simulink model "inverted_pendulum_2dof"  (R2021b)
settings: Solver=ode45  StartTime=0.0  StopTime=10.0  RelTol=1e-3
undefined symbols (not defined in the file): d, F, g, L, M, m, o_0, t_0, v_0, x_0
settings Model: Creator=lenna  LastModifiedBy=lenna

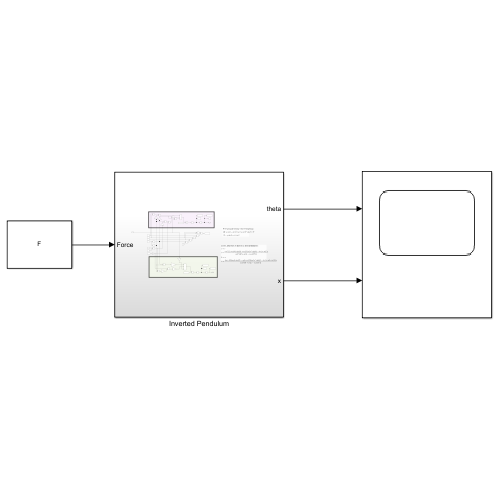
[thumbnail: Simulink's stored preview of the top-level diagram]
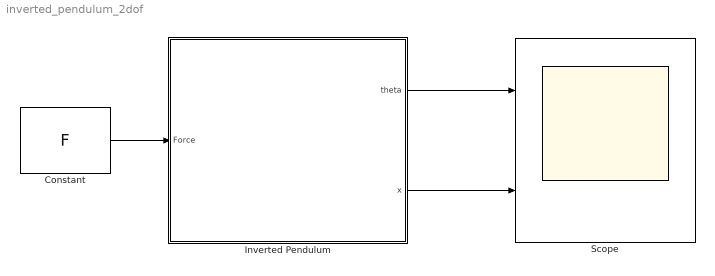
== system inverted_pendulum_2dof ==
  Constant : Constant  Value=F
  Inverted Pendulum : Subsystem
  Scope : Scope  NumInputPorts=2
  wires:
  Constant/1 -> Inverted Pendulum/1(Force)
  Inverted Pendulum/1(theta) -> Scope/1
  Inverted Pendulum/2(x) -> Scope/2

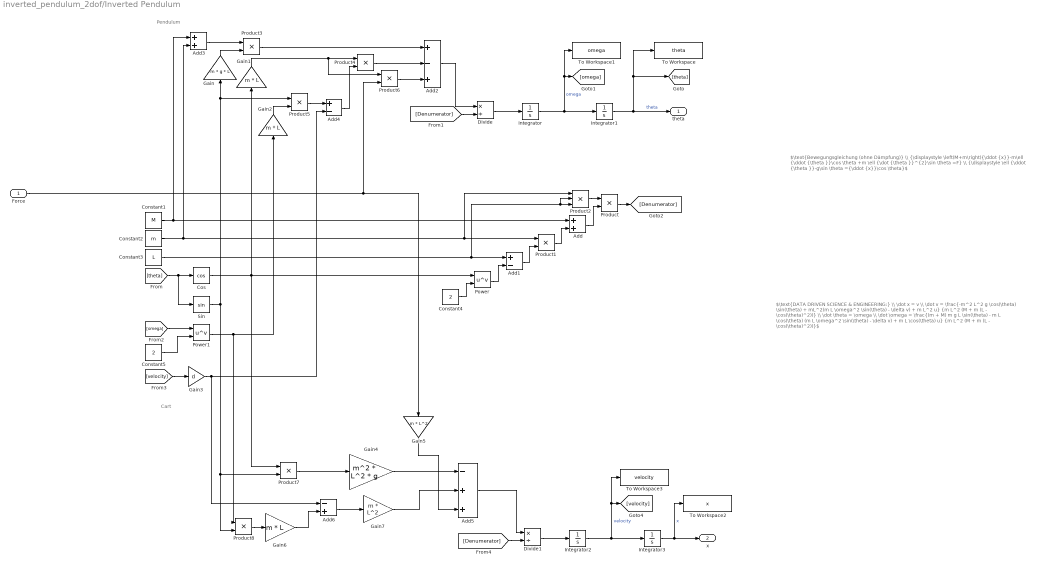
== system inverted_pendulum_2dof/Inverted Pendulum ==
  note: Pendulum
  note: Cart
  note: $\text{DATA DRIVEN SCIENCE & ENGINEERING:} \\ \dot x = v \\ \dot v = \frac{-m^2 L^2 g \cos(\theta) \sin(\theta) + mL^2(m L \omega^2 \sin(\theta) - \delta v) + m L^2 u} {m L^2 (M + m (L - \cos(\theta)^2))} \\ \dot \theta = \omega \\ \dot \omega = \frac{(m + M) m g L \sin(\theta) - m L \cos(\theta) (m L \omega^2 \sin(\theta) - \delta v) + m L \cos(\theta) u} {m L^2 (M + m (L - \cos(\theta)^2))}$
  note: $\text{Bewegungsgleichung (ohne Dämpfung)} \\ {\displaystyle \left(M+m\right){\ddot {x}}-m\ell {\ddot {\theta }}\cos \theta +m \ell {\dot {\theta }}^{2}\sin \theta =F} \\ {\displaystyle \ell {\ddot {\theta }}-g\sin \theta ={\ddot {x}}\cos \theta}$
  Force : Inport
  Add : Sum
  Add1 : Sum  Inputs=+-
  Add2 : Sum  Inputs=+-+
  Add3 : Sum
  Add4 : Sum  Inputs=+-
  Add5 : Sum  Inputs=-++
  Add6 : Sum  Inputs=-+
  Constant1 : Constant  Value=M
  Constant2 : Constant  Value=m
  Constant3 : Constant  Value=L
  Constant4 : Constant  Value=2
  Constant5 : Constant  Value=2
  Cos : Trigonometry  Operator=cos
  Divide : Product  Inputs=*/
  Divide1 : Product  Inputs=*/
  Gain : Gain  Gain=m * g * L
  Gain1 : Gain  Gain=m * L
  Gain2 : Gain  Gain=m * L
  Gain3 : Gain  Gain=d
  Gain4 : Gain  Gain=m^2 * L^2 * g
  Gain5 : Gain  Gain=m * L^2
  Gain6 : Gain  Gain=m * L
  Gain7 : Gain  Gain=m * L^2
  Integrator : Integrator  InitialCondition=o_0
  Integrator1 : Integrator  InitialCondition=t_0
  Integrator2 : Integrator  InitialCondition=v_0
  Integrator3 : Integrator  InitialCondition=x_0
  Power : Math  Operator=pow  SaturateOnIntegerOverflow=on
  Power1 : Math  Operator=pow  SaturateOnIntegerOverflow=on
  Product{,1,3..8} (8 alike) : Product
  Product2 : Product  Inputs=3
  Sin : Trigonometry
  To Workspace : ToWorkspace  VariableName=theta  SampleTime=-1
  To Workspace1 : ToWorkspace  VariableName=omega  SampleTime=-1
  To Workspace2 : ToWorkspace  VariableName=x  SampleTime=-1
  To Workspace3 : ToWorkspace  VariableName=velocity  SampleTime=-1
  theta : Outport
  x : Outport  Port=2
  wires:
  Add2/1 -> Divide/1
  Constant4/1 -> Power/2
  Gain2/1 -> Product5/2
  Integrator3/1 -> x/1, To Workspace2/1  "x"
  [Denumerator] -> Divide/2
  Gain3/1 -> Add4/2, Add6/1
  [theta] -> Sin/1, Cos/1
  Add5/1 -> Divide1/1
  Gain5/1 -> Add5/3
  Gain4/1 -> Add5/1
  Product3/1 -> Add2/1
  Integrator/1 -> To Workspace1/1, [omega], Integrator1/1  "omega"
  Power/1 -> Add1/2
  Sin/1 -> Product8/2, Product7/2, Product5/1, Gain/1
  Gain7/1 -> Add5/2
  Power1/1 -> Gain2/1, Product8/1
  Integrator2/1 -> To Workspace3/1, [velocity], Integrator3/1  "velocity"
  Product/1 -> [Denumerator]
  Add6/1 -> Gain7/1
  Product8/1 -> Gain6/1
  Add/1 -> Product/2
  Cos/1 -> Product7/1, Power/1, Gain1/1
  Constant3/1 -> Product2/2, Product2/3, Add1/1
  Integrator1/1 -> theta/1, [theta], To Workspace/1  "theta"
  Divide1/1 -> Integrator2/1
  Product4/1 -> Add2/2
  Gain/1 -> Product3/2
  Constant1/1 -> Add/1, Add3/1
  Constant2/1 -> Product2/1, Product1/1, Add3/2
  Add1/1 -> Product1/2
  Add3/1 -> Product3/1
  [Denumerator] -> Divide1/2
  Product2/1 -> Product/1
  Gain1/1 -> Product6/1, Product4/1
  Force/1 -> Gain5/1, Product6/2
  Product5/1 -> Add4/1
  Product6/1 -> Add2/3
  Product1/1 -> Add/2
  Product7/1 -> Gain4/1
  Divide/1 -> Integrator/1
  Gain6/1 -> Add6/2
  [omega] -> Power1/1
  Constant5/1 -> Power1/2
  [velocity] -> Gain3/1
  Add4/1 -> Product4/2
